simulink model "model1"  (R2024a)
settings: Solver=VariableStepAuto  StartTime=0.0  StopTime=10.0  RelTol=1e-3
settings Model: Creator=Lenovo  LastModifiedBy=Lenovo

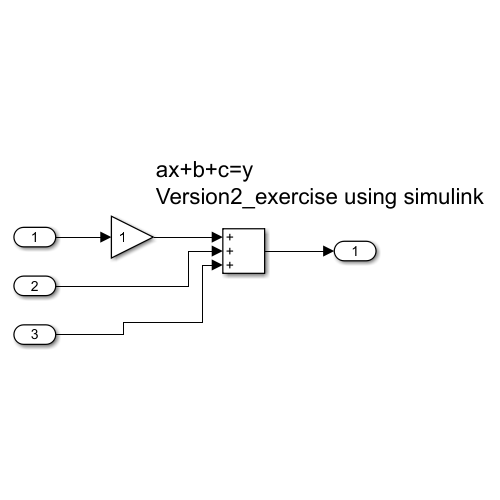
[thumbnail: Simulink's stored preview of the top-level diagram]
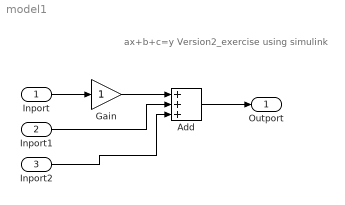
== system model1 ==
  note: ax+b+c=y
      | Version2_exercise using simulink
  Inport : Inport
  Inport1 : Inport  Port=2
  Inport2 : Inport  Port=3
  Add : Sum  Inputs=+++
  Gain : Gain
  Outport : Outport
  wires:
  Inport/1 -> Gain/1
  Gain/1 -> Add/1
  Inport1/1 -> Add/2
  Add/1 -> Outport/1
  Inport2/1 -> Add/3
